simulink model "zad3_kaskada"  (R2018b)
settings: Solver=VariableStepAuto  StartTime=0.0  StopTime=300  RelTol=1e-3
settings Model: Creator=nahla  LastModifiedBy=nahla

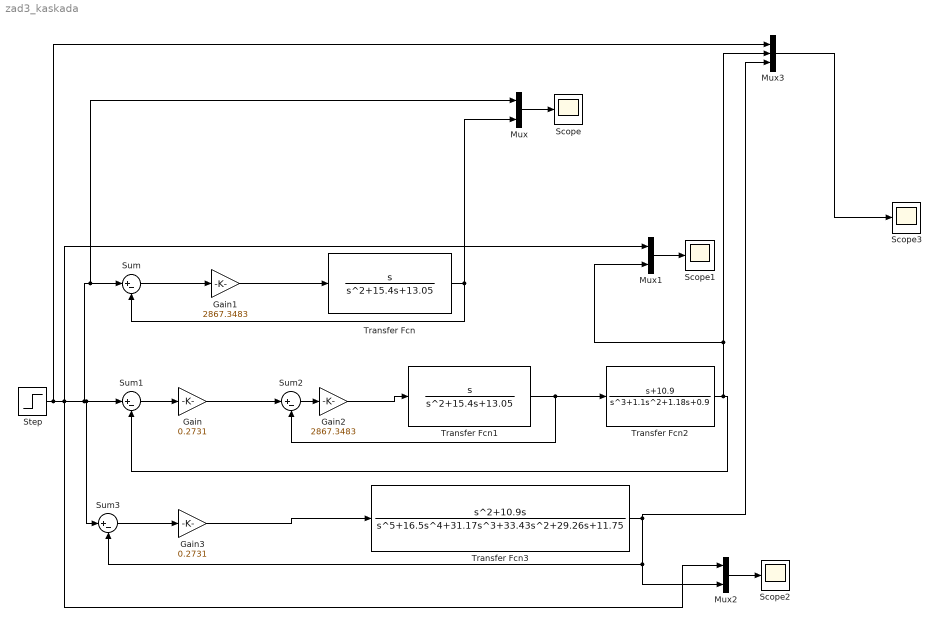
== system zad3_kaskada ==
  Gain : Gain  Gain=0.2731
  Gain1 : Gain  Gain=2867.3483
  Gain2 : Gain  Gain=2867.3483
  Gain3 : Gain  Gain=0.2731
  Mux : Mux  Inputs=2
  Mux1 : Mux  Inputs=2
  Mux2 : Mux  Inputs=2
  Mux3 : Mux  Inputs=3
  Scope{,1..3} (4 alike) : Scope
  Step : Step  SampleTime=0
  Sum{,1..3} (4 alike) : Sum  Inputs=|+-
  Transfer Fcn : TransferFcn  Numerator=[1 0]  Denominator=[1 15.4 13.05]
  Transfer Fcn1 : TransferFcn  Numerator=[1 0]  Denominator=[1 15.4 13.05]
  Transfer Fcn2 : TransferFcn  Numerator=[1 10.9]  Denominator=[1 1.1 1.18 0.9]
  Transfer Fcn3 : TransferFcn  Numerator=[1 10.9 0]  Denominator=[1 16.5 31.17 33.43 29.26 11.75]
  wires:
  Gain/1 -> Sum2/1
  Transfer Fcn3/1 -> Mux2/2, Sum3/2, Mux3/3
  Sum2/1 -> Gain2/1
  Mux1/1 -> Scope1/1
  Sum1/1 -> Gain/1
  Mux/1 -> Scope/1
  Mux2/1 -> Scope2/1
  Step/1 -> Mux3/1, Mux2/1, Mux1/1, Sum3/1, Sum1/1, Mux/1, Sum/1
  Sum3/1 -> Gain3/1
  Sum/1 -> Gain1/1
  Transfer Fcn2/1 -> Mux3/2, Mux1/2, Sum1/2
  Transfer Fcn/1 -> Mux/2, Sum/2
  Gain3/1 -> Transfer Fcn3/1
  Mux3/1 -> Scope3/1
  Gain2/1 -> Transfer Fcn1/1
  Transfer Fcn1/1 -> Sum2/2, Transfer Fcn2/1
  Gain1/1 -> Transfer Fcn/1
